simulink model "F28379D_IPC_CPU2_2020a_pp"  (R2021a)
settings: Solver=FixedStepAuto  StartTime=0.0  StopTime=inf  FixedStep=0.001  RelTol=1e-3  EnableMultiTasking=on
PostLoadFcn:
  | c2000demoscallback(1);
model workspace (MAT data in the model file):
  encoderResolution = 2000
  hallOffset = '0.5'
  indexOffset = 850
  polePairs = '4'
undefined symbols (not defined in the file): angdiff, C28x, CPU1, CPU2, lh
libraries: c2837xDlib x2, c280xlib x1, c2000lib x1, canmsglib x1
settings Model: ExtModeTrigDuration=8  Creator=The MathWorks, Inc.  LastModifiedBy=Jamie
settings SolverCC: AlgebraicLoopSolver=TrustRegion  AutoInsertRateTranBlk=on
settings DataIOCC: LimitDataPoints=on  SaveFormat=Array  SaveOutput=off  SaveTime=off  ReturnWorkspaceOutputs=off
settings OptimizationCC: DefaultUnderspecifiedDataType=single  OptimizeBlockIOStorage=off  BufferReuse=off  GlobalBufferReuse=off  ExpressionFolding=off  ExpressionDepthLimit=2147483647  LocalBlockOutputs=off  InitFltsAndDblsToZero=on  NoFixptDivByZeroProtection=on  EfficientFloat2IntCast=on  EfficientMapNaN2IntZero=off  LifeSpan=Inf  MaxStackSize=512  OptimizeDataStoreBuffers=off  BusAssignmentInplaceUpdate=off  EfficientTunableParamExpr=on
settings DebuggingCC: ReadBeforeWriteMsg=DisableAll  WriteAfterWriteMsg=DisableAll  WriteAfterReadMsg=DisableAll  CheckSSInitialOutputMsg=off  UnderspecifiedInitializationDetection=Classic  MergeDetectMultiDrivingBlocksExec=none  SignalResolutionControl=TryResolveAllWithWarning  SolverPrmCheckMsg=warning  InheritedTsInSrcMsg=none  MultiTaskDSMMsg=none  MultiTaskCondExecSysMsg=none  TasksWithSamePriorityMsg=none  SigSpecEnsureSampleTimeMsg=none  IntegerOverflowMsg=none  ParameterPrecisionLossMsg=none  FcnCallInpInsideContextMsg=warning  AllowSymbolicDim=off  StateNameClashWarn=warning  SFUnexpectedBacktrackingDiag=warning  SFNoUnconditionalDefaultTransitionDiag=warning  SFExecutionAtInitializationDiag=none  SFMachineParentedDataDiag=warning  IntegerSaturationMsg=none  ArithmeticOperatorsInVariantConditions=warning
settings HardwareCC: ProdBitPerChar=16  ProdBitPerInt=16  ProdBitPerPointer=32  ProdBitPerSizeT=32  ProdBitPerPtrDiffT=32  ProdLargestAtomicInteger=Integer  ProdLargestAtomicFloat=None  ProdWordSize=16  ProdLongLongMode=on  ProdHWDeviceType=Texas Instruments->C2000  TargetBitPerChar=16  TargetBitPerInt=16  TargetBitPerPointer=16  TargetLargestAtomicInteger=Integer  TargetIntDivRoundTo=Zero  TargetEndianess=LittleEndian  TargetWordSize=16  TargetHWDeviceType=TI C2000
settings ModelReferenceCC: PropagateSignalLabelsOutOfModel=off
settings SFSimCC: SimUseLocalCustomCode=off  MATLABDynamicMemAlloc=off  CustomCodeUndefinedFunction=UseInterfaceOnly
settings RTWCC: SystemTargetFile=ert.tlc  HardwareBoard=TI Delfino F2837xD  TemplateMakefile=ert_default_tmf  GenerateReport=on  RTWUseLocalCustomCode=off  Toolchain=Texas Instruments Code Composer Studio (C2000)  IncludeHyperlinkInReport=on  LaunchReport=on  GenerateTraceInfo=on  GenerateTraceReport=on  GenerateTraceReportSl=on  GenerateTraceReportSf=on  GenerateTraceReportEml=on
settings CodeAppCC: IgnoreCustomStorageClasses=off  CustomSymbolStrType=$N$R$M  StateflowObjectComments=on  InternalIdentifier=Classic
settings ERTTargetCC: CodeReplacementLibrary=TI C28x  MultiwordLength=2048  SupportContinuousTime=on  ConvertIfToSwitch=off  SuppressUnreachableDefaultCases=off  MemSecPackage=tic2000demospkg
settings ConfigComp: CovMetricSettings=dw  CovSaveCumulativeToWorkspaceVar=on  CovSaveSingleToWorkspaceVar=on  CovExternalEMLEnable=off  CovSFcnEnable=off

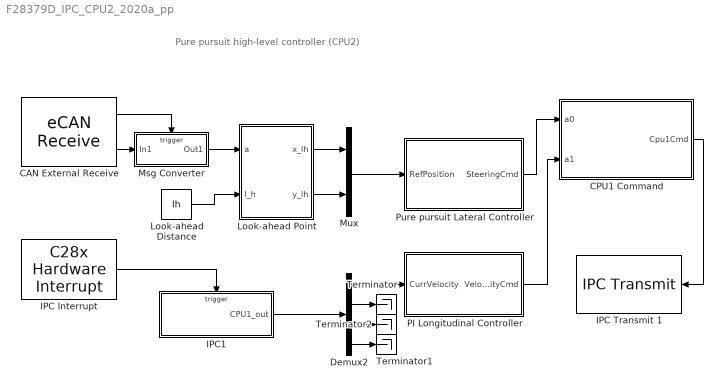
== system F28379D_IPC_CPU2_2020a_pp ==
  note: Pure pursuit high-level controller (CPU2)
  CAN External Receive : c280xlib/eCAN Receive  chipFamily=C280x  useModule=eCAN_B  mailboxNo=0  messageID=bin2dec('1')  messageType=Standard (11-bit identifier)  sampleTime=0.005  dataType=CAN_MESSAGE_TYPE  initValue=0  outputMessageLength=off  outputMessageTimeStamp=off  postInterrupt=off  interruptLine=0
      settings: SourceProductBaseCode=TIC2000
  CPU1 Command : MATLAB Function  TreatAsAtomicUnit=on  RTWFcnName=uint16Tofloat16  RTWFileName=uint16Tofloat16
      settings: RTWFileNameOpts=User specified
  Demux2 : Demux
  IPC Interrupt : c2000lib/Scheduling/C28x Hardware Interrupt  irqnumbers=[1]  pienumbers=[14]  irqpriorities=[29]  irqpreempts=[1]  showinput=off  dspchiptype=C280X
      settings: SourceProductBaseCode=TIC2000
  IPC Transmit 1 : c2837xDlib/IPC Transmit  blkParamProc=F2837x  SelectDestination=C28x (CPU1/CPU2)  SelectChannel=1  EnableBlocking=off
      settings: SourceProductBaseCode=TIC2000
  IPC1 : Subsystem  TreatAsAtomicUnit=on
  Look-ahead Distance : Constant  Value=lh  OutDataTypeStr=single
  Look-ahead Point : MATLAB Function  TreatAsAtomicUnit=on
  Msg Converter : Subsystem  TreatAsAtomicUnit=on
  Mux : Mux  Inputs=2
  PI Longitudinal Controller : Subsystem
  Pure pursuit Lateral Controller : Subsystem
  Terminator : Terminator
  Terminator1 : Terminator
  Terminator2 : Terminator
  wires:
  CAN External Receive/1 -> Msg Converter/Trigger
  CAN External Receive/2 -> Msg Converter/1(In1)
  IPC Interrupt/1 -> IPC1/Trigger
  Look-ahead Point/1(x_lh) -> Mux/1
  Look-ahead Distance/1 -> Look-ahead Point/2(l_h)
  Mux/1 -> Pure pursuit Lateral Controller/1(RefPosition)
  CPU1 Command/1(Cpu1Cmd) -> IPC Transmit 1/1
  IPC1/1(CPU1_out) -> Demux2/1
  Look-ahead Point/2(y_lh) -> Mux/2
  Demux2/1 -> PI Longitudinal Controller/1(CurrVelocity)
  Pure pursuit Lateral Controller/1(SteeringCmd) -> CPU1 Command/1(a0)
  PI Longitudinal Controller/1(VelocityCmd) -> CPU1 Command/2(a1)
  Demux2/2 -> Terminator/1
  Demux2/3 -> Terminator2/1
  Demux2/4 -> Terminator1/1
  Msg Converter/1(Out1) -> Look-ahead Point/1(a)

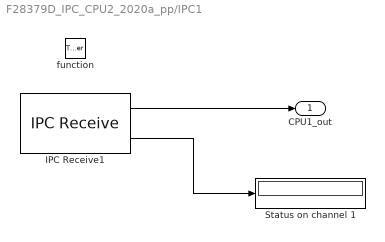
== system F28379D_IPC_CPU2_2020a_pp/IPC1 ==
  function : TriggerPort  TriggerType=function-call  VariantControl=Variant
  IPC Receive1 : c2837xDlib/IPC Receive  blkParamProc=F2837x  SelectSource=C28x (CPU1/CPU2)  SelectChannel=1  DataType=single  DataLength=4  EnableBlocking=off  SampleTime=-1
      settings: SourceProductBaseCode=TIC2000
  Status on channel 1 : Display
  CPU1_out : Outport
  wires:
  IPC Receive1/2 -> Status on channel 1/1
  IPC Receive1/1 -> CPU1_out/1

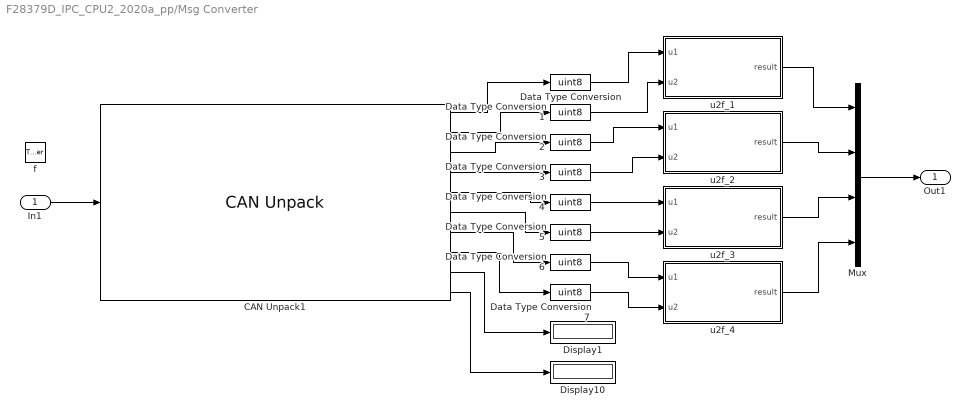
== system F28379D_IPC_CPU2_2020a_pp/Msg Converter ==
  In1 : Inport
  f : TriggerPort  TriggerType=function-call  VariantControl=Variant
  CAN Unpack1 : canmsglib/CAN Unpack  MsgList=(none)  MsgName=CAN Msg  MsgIDType=Standard (11-bit identifier)  MsgIdentifier=bin2dec('1')  MsgLength=8  SignalInfo={ 'Signal1', '0', '8', 'LE', 'unsigned', 'Standard', '0', '1', '0', '0', '255'; 'Signal2', '8', '8', 'LE', 'unsigned', 'Standard', '0', '1', '0', '0', '255'; 'Signal3', '16', '8', 'LE', 'unsigned', 'Standard', '0', '1', '0', '0', '255'; 'Signal4', '24', '8', 'LE', 'unsigned', 'Standard', '0', '1', '0', '0', '255'; 'Signal5', '32', '8', 'LE', 'unsigned', 'Standard', '0', '1', '0', '0', '255'; 'Signal6', '40', '8', 'LE', 'unsigned', 'Standard', '0', '1', '0', '0', '255'; 'Signal7', '48', '8', 'LE', 'unsigned', 'Standard', '0', '1', '0', '0', '255'; 'Signal8', '56', '8', 'LE', 'unsigned', 'Standard', '0', '1', '0', '0', '255' }  IDPort=off  TimestampPort=off  ErrorPort=off  RemotePort=off  LengthPort=on  StatusPort=on  ApplyMinMax=off
      settings: SourceProductBaseCode=ME,XP,VN
  Data Type Conversion{,1..7} (8 alike) : DataTypeConversion  OutDataTypeStr=uint8
  Display1 : Display
  Display10 : Display
  Mux : Mux
  u2f_1 : MATLAB Function  TreatAsAtomicUnit=on  RTWFcnName=uint16Tofloat16  RTWFileName=uint16Tofloat16
      settings: RTWFileNameOpts=User specified
  u2f_2 : MATLAB Function  TreatAsAtomicUnit=on  RTWFcnName=uint16Tofloat16  RTWFileName=uint16Tofloat16
      settings: RTWFileNameOpts=User specified
  u2f_3 : MATLAB Function  TreatAsAtomicUnit=on  RTWFcnName=uint16Tofloat16  RTWFileName=uint16Tofloat16
      settings: RTWFileNameOpts=User specified
  u2f_4 : MATLAB Function  TreatAsAtomicUnit=on  RTWFcnName=uint16Tofloat16  RTWFileName=uint16Tofloat16
      settings: RTWFileNameOpts=User specified
  Out1 : Outport
  wires:
  In1/1 -> CAN Unpack1/1
  CAN Unpack1/9 -> Display1/1
  CAN Unpack1/10 -> Display10/1
  CAN Unpack1/1 -> Data Type Conversion/1
  CAN Unpack1/2 -> Data Type Conversion1/1
  CAN Unpack1/3 -> Data Type Conversion2/1
  CAN Unpack1/4 -> Data Type Conversion3/1
  CAN Unpack1/5 -> Data Type Conversion4/1
  CAN Unpack1/6 -> Data Type Conversion5/1
  CAN Unpack1/7 -> Data Type Conversion6/1
  CAN Unpack1/8 -> Data Type Conversion7/1
  Data Type Conversion/1 -> u2f_1/1(u1)
  Data Type Conversion1/1 -> u2f_1/2(u2)
  Data Type Conversion2/1 -> u2f_2/1(u1)
  Data Type Conversion3/1 -> u2f_2/2(u2)
  Data Type Conversion4/1 -> u2f_3/1(u1)
  Data Type Conversion5/1 -> u2f_3/2(u2)
  Data Type Conversion6/1 -> u2f_4/1(u1)
  Data Type Conversion7/1 -> u2f_4/2(u2)
  Mux/1 -> Out1/1
  u2f_1/1(result) -> Mux/1
  u2f_2/1(result) -> Mux/2
  u2f_3/1(result) -> Mux/3
  u2f_4/1(result) -> Mux/4

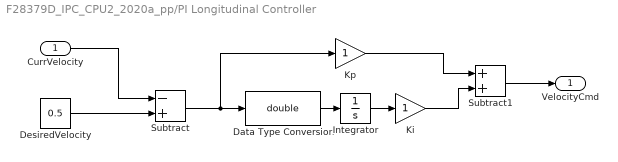
== system F28379D_IPC_CPU2_2020a_pp/PI Longitudinal Controller ==
  CurrVelocity : Inport
  Data Type Conversion : DataTypeConversion  OutDataTypeStr=double
  DesiredVelocity : Constant  Value=0.5  OutDataTypeStr=single
  Integrator : Integrator
  Ki : Gain  OutDataTypeStr=single
  Kp : Gain  OutDataTypeStr=single
  Subtract : Sum  Inputs=-+  OutDataTypeStr=single
  Subtract1 : Sum  AccumDataTypeStr=single
  VelocityCmd : Outport
  wires:
  Subtract1/1 -> VelocityCmd/1
  DesiredVelocity/1 -> Subtract/2
  Ki/1 -> Subtract1/2
  Subtract/1 -> Kp/1, Data Type Conversion/1
  Integrator/1 -> Ki/1
  Kp/1 -> Subtract1/1
  CurrVelocity/1 -> Subtract/1
  Data Type Conversion/1 -> Integrator/1

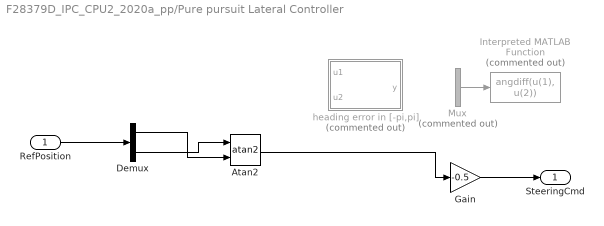
== system F28379D_IPC_CPU2_2020a_pp/Pure pursuit Lateral Controller ==
  RefPosition : Inport
  Atan2 : Trigonometry  Operator=atan2
  Demux : Demux  Outputs=2
  Gain : Gain  Gain=-0.5
  Interpreted MATLAB Function : MATLABFcn  Commented=on  MATLABFcn=angdiff(u(1), u(2))  OutputSignalType=real
  Mux : Mux  Commented=on  Inputs=2
  heading error in [-pi,pi] : MATLAB Function  Commented=on  TreatAsAtomicUnit=on
  SteeringCmd : Outport
  wires:
  Demux/2 -> Atan2/1
  Demux/1 -> Atan2/2
  Mux/1 -> Interpreted MATLAB Function/1
  Gain/1 -> SteeringCmd/1
  RefPosition/1 -> Demux/1
  Atan2/1 -> Gain/1

== matlab function F28379D_IPC_CPU2_2020a_pp/Msg Converter/u2f_2 ==
  data: u1 input; result output; u2 input
function result = uint16Tofloat16(u1, u2)

% hex2bin(u1) % high 8-bit
% hex2bin(u2) % low 8-bit

%% Return a 16-bit value
% a = uint16(u1);
% b = uint16(u2);
% c = uint16(256*a + b);

%% Return a 16-bit half precision float
a = uint16(u1);
b = uint16(u2);
c = uint16(256*a + b);

% Get sign bit
sign_bit = bitsrl(c, 15);
sign_bit = uint8(sign_bit);

% Get exponent
exponent = bitand(c, 0b0111110000000000);
exponent = bitsrl(exponent, 10);
exponent = single(exponent);

% Get significantbits
significant = bitand(c, 0b0000001111111111);
significant = uint16(significant);

if exponent == 0
    if(significant == 0)
        result = single(0.0);
    else
        if(sign_bit == 0) % positive
            result = 2^(-14) * get_significant(significant);
        else % negative
            result = -2^(-14)* get_significant(significant);
        end
    end
elseif exponent == 31 % 0x1f, infinity number
    % the maximum number is 65504
    result = single(65504 + 1); % 
else
    % exponent is btw 0b00001 and 0b11110
    if(sign_bit == 0) % positive
        result = 2^(exponent-15) * (1 + get_significant(significant));
    else % negative
        result = -2^(exponent-15) * (1 + get_significant(significant));
    end
 
end

function significant_result = get_significant(x)
    m = x;
    n = 10;
    significant_result = 0;
    for i = 1:10
        if bitand(m, 0x0001) == 0x0001
            significant_result = significant_result + 2^(-n);
        end
        n = n-1;
        m = bitsrl(x, i);
    end  
    significant_result = single(significant_result);
end
    
end % function end

== matlab function F28379D_IPC_CPU2_2020a_pp/Msg Converter/u2f_3 ==
  data: u1 input; result output; u2 input
function result = uint16Tofloat16(u1, u2)

% hex2bin(u1) % high 8-bit
% hex2bin(u2) % low 8-bit

%% Return a 16-bit value
% a = uint16(u1);
% b = uint16(u2);
% c = uint16(256*a + b);

%% Return a 16-bit half precision float
a = uint16(u1);
b = uint16(u2);
c = uint16(256*a + b);

% Get sign bit
sign_bit = bitsrl(c, 15);
sign_bit = uint8(sign_bit);

% Get exponent
exponent = bitand(c, 0b0111110000000000);
exponent = bitsrl(exponent, 10);
exponent = single(exponent);

% Get significantbits
significant = bitand(c, 0b0000001111111111);
significant = uint16(significant);

if exponent == 0
    if(significant == 0)
        result = single(0.0);
    else
        if(sign_bit == 0) % positive
            result = 2^(-14) * get_significant(significant);
        else % negative
            result = -2^(-14)* get_significant(significant);
        end
    end
elseif exponent == 31 % 0x1f, infinity number
    % the maximum number is 65504
    result = single(65504 + 1); % 
else
    % exponent is btw 0b00001 and 0b11110
    if(sign_bit == 0) % positive
        result = 2^(exponent-15) * (1 + get_significant(significant));
    else % negative
        result = -2^(exponent-15) * (1 + get_significant(significant));
    end
 
end

function significant_result = get_significant(x)
    m = x;
    n = 10;
    significant_result = 0;
    for i = 1:10
        if bitand(m, 0x0001) == 0x0001
            significant_result = significant_result + 2^(-n);
        end
        n = n-1;
        m = bitsrl(x, i);
    end  
    significant_result = single(significant_result);
end
    
end % function end

== matlab function F28379D_IPC_CPU2_2020a_pp/Msg Converter/u2f_4 ==
  data: u1 input; result output; u2 input
function result = uint16Tofloat16(u1, u2)

% hex2bin(u1) % high 8-bit
% hex2bin(u2) % low 8-bit

%% Return a 16-bit value
% a = uint16(u1);
% b = uint16(u2);
% c = uint16(256*a + b);

%% Return a 16-bit half precision float
a = uint16(u1);
b = uint16(u2);
c = uint16(256*a + b);

% Get sign bit
sign_bit = bitsrl(c, 15);
sign_bit = uint8(sign_bit);

% Get exponent
exponent = bitand(c, 0b0111110000000000);
exponent = bitsrl(exponent, 10);
exponent = single(exponent);

% Get significantbits
significant = bitand(c, 0b0000001111111111);
significant = uint16(significant);

if exponent == 0
    if(significant == 0)
        result = single(0.0);
    else
        if(sign_bit == 0) % positive
            result = 2^(-14) * get_significant(significant);
        else % negative
            result = -2^(-14)* get_significant(significant);
        end
    end
elseif exponent == 31 % 0x1f, infinity number
    % the maximum number is 65504
    result = single(65504 + 1); % 
else
    % exponent is btw 0b00001 and 0b11110
    if(sign_bit == 0) % positive
        result = 2^(exponent-15) * (1 + get_significant(significant));
    else % negative
        result = -2^(exponent-15) * (1 + get_significant(significant));
    end
 
end

function significant_result = get_significant(x)
    m = x;
    n = 10;
    significant_result = 0;
    for i = 1:10
        if bitand(m, 0x0001) == 0x0001
            significant_result = significant_result + 2^(-n);
        end
        n = n-1;
        m = bitsrl(x, i);
    end  
    significant_result = single(significant_result);
end
    
end % function end

== matlab function F28379D_IPC_CPU2_2020a_pp/Msg Converter/u2f_1 ==
  data: u1 input; result output; u2 input
function result = uint16Tofloat16(u1, u2)

% hex2bin(u1) % high 8-bit
% hex2bin(u2) % low 8-bit

%% Return a 16-bit value
% a = uint16(u1);
% b = uint16(u2);
% c = uint16(256*a + b);

%% Return a 16-bit half precision float
a = uint16(u1);
b = uint16(u2);
c = uint16(256*a + b);

% Get sign bit
sign_bit = bitsrl(c, 15);
sign_bit = uint8(sign_bit);

% Get exponent
exponent = bitand(c, 0b0111110000000000);
exponent = bitsrl(exponent, 10);
exponent = single(exponent);

% Get significantbits
significant = bitand(c, 0b0000001111111111);
significant = uint16(significant);

if exponent == 0
    if(significant == 0)
        result = single(0.0);
    else
        if(sign_bit == 0) % positive
            result = 2^(-14) * get_significant(significant);
        else % negative
            result = -2^(-14)* get_significant(significant);
        end
    end
elseif exponent == 31 % 0x1f, infinity number
    % the maximum number is 65504
    result = single(65504 + 1); % 
else
    % exponent is btw 0b00001 and 0b11110
    if(sign_bit == 0) % positive
        result = 2^(exponent-15) * (1 + get_significant(significant));
    else % negative
        result = -2^(exponent-15) * (1 + get_significant(significant));
    end
 
end

function significant_result = get_significant(x)
    m = x;
    n = 10;
    significant_result = 0;
    for i = 1:10
        if bitand(m, 0x0001) == 0x0001
            significant_result = significant_result + 2^(-n);
        end
        n = n-1;
        m = bitsrl(x, i);
    end  
    significant_result = single(significant_result);
end
    
end % function end

== matlab function F28379D_IPC_CPU2_2020a_pp/Look-ahead Point ==
  data: x_lh output; y_lh output; a input; l_h input
function [x_lh,y_lh] = fcn(a, l_h)


a_0 = a[1];
a_1 = a[2];
a_2 = a[3];
a_3 = a[4];

% input four parameter, look_ahead distance 
i = 0;
   %in the loop, find a point distance to the car = look ahead distance 
while(1)
    x_t = l_h - i; % start from x=l_h, y=0,
    y_t = a_3*x_t^3 + a_2*x_t^2 + a_1*x_t + a_0; %(x_t, y_t) points on the curve
    
    d_t = sqrt(x_t^2 + y_t^2);
    if(x_t <= 0.01)
        x_lh = single(l_h); %if no pointds found, x_t = 0, no look ahead point found, go straight ahead
        y_lh = single(0.0);
        break
    else
        if(abs(d_t - l_h) <= 0.01)%if find the look ahead point ,break and return
            x_lh = single(x_t);
            y_lh = single(y_t);
            break;  
        else
            i = i + 0.01;
        end
    end

end

== matlab function F28379D_IPC_CPU2_2020a_pp/CPU1 Command ==
  data: a0 input; Cpu1Cmd output; a1 input
function Cpu1Cmd = cpu1_array(a0, a1)

Cpu1Cmd = [a0, a1, 0, 0];
    
end % function end

== matlab function F28379D_IPC_CPU2_2020a_pp/Pure pursuit Lateral Controller/heading error in [-pi,pi] ==
  data: u1 input; y output; u2 input
function y = fcn(u1, u2)
    du = u1 - u2;
    while (du > pi)
        du = du - 2*pi
    end
    
    while (du < -pi)
        du = du + 2*pi
    end
y = du;
